simulink model "pendule_inv_capteur_etu"  (R2022a)
settings: Solver=VariableStepAuto  StartTime=0.0  StopTime=10.0  RelTol=1e-3
values from neighbouring files (symbols this model uses):
  g = 9.81    [simu_pendule_inv_capteur_etu.m]    (also in simu_pendule_inv_echant_etu.m; simu_pendule_inv_etu.m)
  K = [10 1]    [simu_pendule_inv_capteur_etu.m]    (also in simu_pendule_inv_echant_etu.m = [30 10]; simu_pendule_inv_etu.m = [30 10])
  l = 10    [simu_pendule_inv_capteur_etu.m]    (also in simu_pendule_inv_echant_etu.m; simu_pendule_inv_etu.m)
  ue = 0    [simu_pendule_inv_capteur_etu.m]    (also in simu_pendule_inv_echant_etu.m; simu_pendule_inv_etu.m)
  x0 = [pi/20 0]'    [simu_pendule_inv_capteur_etu.m]    (also in simu_pendule_inv_echant_etu.m; simu_pendule_inv_etu.m = [pi/10 0]')
  xe = [0 0]'    [simu_pendule_inv_capteur_etu.m]    (also in simu_pendule_inv_echant_etu.m; simu_pendule_inv_etu.m)
settings Model: Creator=nauchere  LastModifiedBy=nauchere

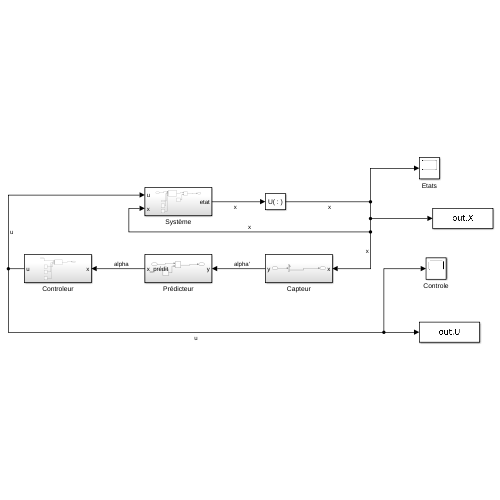
[thumbnail: Simulink's stored preview of the top-level diagram]
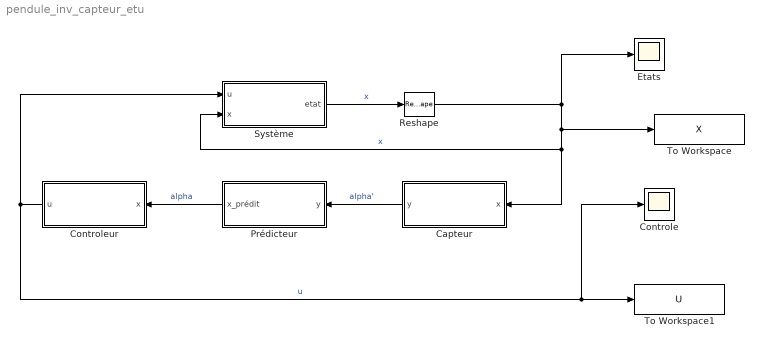
== system pendule_inv_capteur_etu ==
  Capteur : Subsystem
  Controle : Scope
  Controleur : Subsystem
  Etats : Scope
  Prédicteur : Subsystem
  Reshape : Reshape
  Système : Subsystem
  To Workspace : ToWorkspace  VariableName=X  SaveFormat=Timeseries  SampleTime=-1
  To Workspace1 : ToWorkspace  VariableName=U  SaveFormat=Timeseries  SampleTime=-1
  wires:
  Prédicteur/1(x_prédit) -> Controleur/1(x)  "alpha"
  Capteur/1(y) -> Prédicteur/1(y)  "alpha'"
  Controleur/1(u) -> Système/1(u), Controle/1, To Workspace1/1  "u"
  Système/1(etat) -> Reshape/1  "x"
  Reshape/1 -> Système/2(x), Capteur/1(x), To Workspace/1, Etats/1  "x"

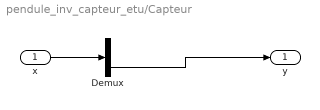
== system pendule_inv_capteur_etu/Capteur ==
  x : Inport
  Demux : Demux  Outputs=2
  y : Outport
  wires:
  x/1 -> Demux/1
  Demux/2 -> y/1

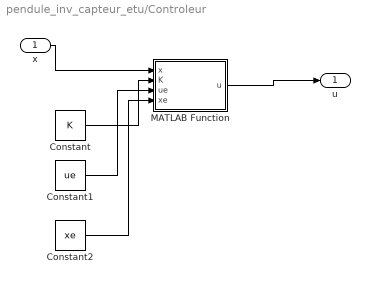
== system pendule_inv_capteur_etu/Controleur ==
  x : Inport
  Constant : Constant  Value=K  VectorParams1D=off
  Constant1 : Constant  Value=ue
  Constant2 : Constant  Value=xe  VectorParams1D=off
  MATLAB Function : MATLAB Function  TreatAsAtomicUnit=on
  u : Outport
  wires:
  Constant2/1 -> MATLAB Function/4(xe)
  MATLAB Function/1(u) -> u/1
  Constant/1 -> MATLAB Function/2(K)
  x/1 -> MATLAB Function/1(x)
  Constant1/1 -> MATLAB Function/3(ue)

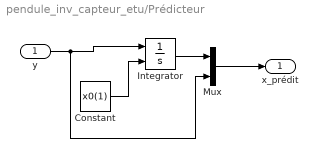
== system pendule_inv_capteur_etu/Prédicteur ==
  y : Inport
  Constant : Constant  Value=x0(1)
  Integrator : Integrator  InitialConditionSource=external
  Mux : Mux  Inputs=2
  x_prédit : Outport
  wires:
  Constant/1 -> Integrator/2
  Mux/1 -> x_prédit/1
  Integrator/1 -> Mux/1
  y/1 -> Mux/2, Integrator/1

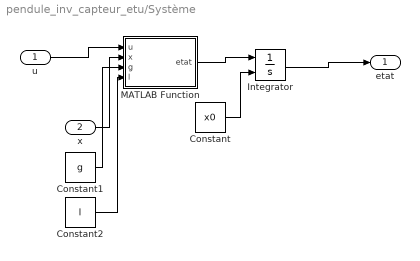
== system pendule_inv_capteur_etu/Système ==
  u : Inport
  x : Inport  Port=2
  Constant : Constant  Value=x0  VectorParams1D=off
  Constant1 : Constant  Value=g
  Constant2 : Constant  Value=l
  Integrator : Integrator  InitialConditionSource=external
  MATLAB Function : MATLAB Function  TreatAsAtomicUnit=on
  etat : Outport
  wires:
  Integrator/1 -> etat/1
  MATLAB Function/1(etat) -> Integrator/1
  u/1 -> MATLAB Function/1(u)
  x/1 -> MATLAB Function/2(x)
  Constant2/1 -> MATLAB Function/4(l)
  Constant/1 -> Integrator/2
  Constant1/1 -> MATLAB Function/3(g)

== matlab function pendule_inv_capteur_etu/Controleur/MATLAB Function ==
  data: x input; u output; K input; ue input; xe input
function u = fcn(x, K, ue, xe)

u = ue + K*(x - xe);
end

== matlab function pendule_inv_capteur_etu/Système/MATLAB Function ==
  data: u input; etat output; x input; g input; l input
function etat = fcn(u,x, g, l)
    x1_p = x(2);
    x2_p = (g/l)*sin(x(1)) - (cos(x(1))*u)/l;
etat = [x1_p x2_p]';
end
